simulink model "Cpchara"  (Simulink 7.4)
settings: Solver=ode45  StartTime=0.0  StopTime=100  RelTol=1e-3
libraries: simulink x3
settings Model: Creator=Balaji  LastModifiedBy=ss
settings DebuggingCC: StrictBusMsg=ErrorLevel1

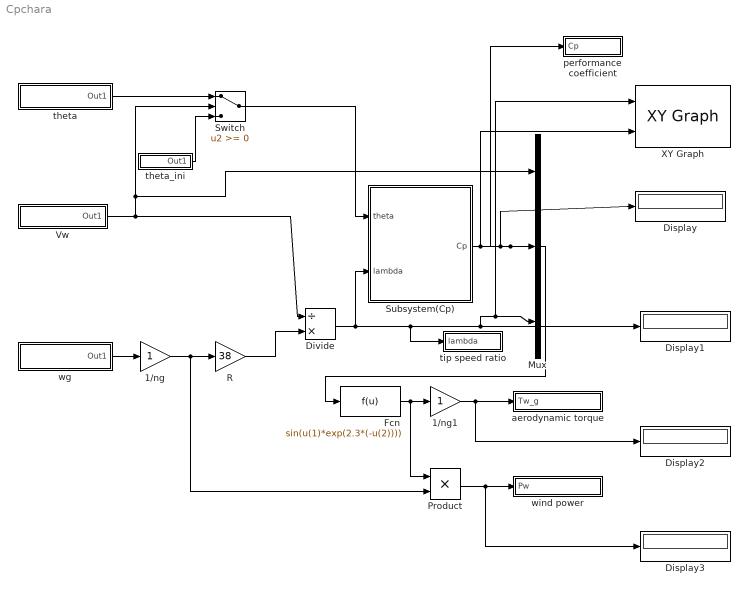
== system Cpchara ==
  1/ng : Gain  ParameterDataType=fixdt(1, 16)  ParameterScaling=2^0  OutDataType=fixdt(1, 16)  OutScaling=2^0
  1/ng1 : Gain  ParameterDataType=fixdt(1, 16)  ParameterScaling=2^0  OutDataType=fixdt(1, 16)  OutScaling=2^0
  Display{,1..3} (4 alike) : Display
  Divide : Product  Inputs=/*  OutDataType=fixdt(1, 16)  OutScaling=2^-10
  Fcn : Fcn  Expr=sin(u(1)*exp(2.3*(-u(2))))
  Mux : Mux  Inputs=3
  Product : Product  OutDataType=fixdt(1, 16)  OutScaling=2^0  RndMeth=Zero
  R : Gain  Gain=38  ParameterDataType=fixdt(1, 16)  ParameterScaling=2^0  OutDataType=fixdt(1, 16)  OutScaling=2^0
  Subsystem(Cp) : Subsystem
  Switch : Switch  OutDataType=fixdt(1, 16)  OutScaling=2^0  SampleTime=5
  Vw : Subsystem
  XY Graph : simulink/Sinks/XY Graph  SystemSampleTime=-1  xmin=2  xmax=16  ymin=0  ymax=0.5  st=0.05
  aerodynamic torque : Subsystem
  performance coefficient : Subsystem
  theta : Subsystem
  theta_ini : Subsystem
  tip speed ratio : Subsystem
  wg : Subsystem
  wind power : Subsystem
  wires:
  wg/1(Out1) -> 1/ng/1
  1/ng/1 -> R/1, Product/2
  Vw/1(Out1) -> Divide/1, Switch/2, Mux/1
  R/1 -> Divide/2
  theta/1(Out1) -> Switch/1
  theta_ini/1(Out1) -> Switch/3
  Switch/1 -> Subsystem(Cp)/1(theta)
  Divide/1 -> tip speed ratio/1(lambda), Display1/1, Mux/3, XY Graph/1, Subsystem(Cp)/2(lambda)
  Mux/1 -> Fcn/1
  Fcn/1 -> 1/ng1/1, Product/1
  1/ng1/1 -> aerodynamic torque/1(Tw_g), Display2/1
  Product/1 -> Display3/1, wind power/1(Pw)
  Subsystem(Cp)/1(Cp) -> Display/1, performance coefficient/1(Cp), Mux/2, XY Graph/2

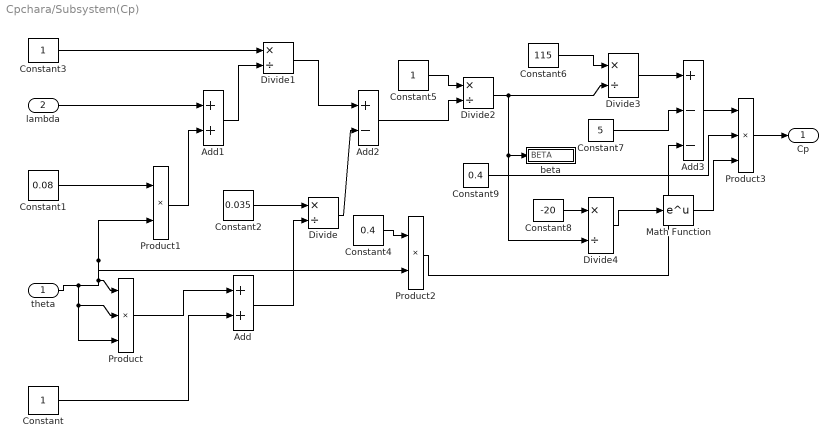
== system Cpchara/Subsystem(Cp) ==
  theta : Inport  OutDataType=fixdt(1, 16)  OutScaling=2^0
  lambda : Inport  Port=2  OutDataType=fixdt(1, 16)  OutScaling=2^0
  Add : Sum  OutDataType=fixdt(1, 16)  OutScaling=2^-10
  Add1 : Sum  OutDataType=fixdt(1, 16)  OutScaling=2^-10
  Add2 : Sum  Inputs=+-  OutDataType=fixdt(1, 16)  OutScaling=2^-10
  Add3 : Sum  Inputs=+--  OutDataType=fixdt(1, 16)  OutScaling=2^-10
  Constant : Constant  OutDataType=fixdt(1, 16)  OutScaling=2^0
  Constant1 : Constant  Value=0.08  OutDataType=fixdt(1, 16)  OutScaling=2^0
  Constant2 : Constant  Value=0.035  OutDataType=fixdt(1, 16)  OutScaling=2^0
  Constant3 : Constant  OutDataType=fixdt(1, 16)  OutScaling=2^0
  Constant4 : Constant  Value=0.4  OutDataType=fixdt(1, 16)  OutScaling=2^0
  Constant5 : Constant  OutDataType=fixdt(1, 16)  OutScaling=2^0
  Constant6 : Constant  Value=115  OutDataType=fixdt(1, 16)  OutScaling=2^0
  Constant7 : Constant  Value=5  OutDataType=fixdt(1, 16)  OutScaling=2^0
  Constant8 : Constant  Value=-20  OutDataType=fixdt(1, 16)  OutScaling=2^0
  Constant9 : Constant  Value=0.4  OutDataType=fixdt(1, 16)  OutScaling=2^0
  Divide{,1..4} (5 alike) : Product  Inputs=*/  OutDataType=fixdt(1, 16)  OutScaling=2^-10
  Math Function : Math  OutDataType=fixdt(1, 16)  OutScaling=2^0  SaturateOnIntegerOverflow=on
  Product : Product  Inputs=3  OutDataType=fixdt(1, 16)  OutScaling=2^0  RndMeth=Zero
  Product1 : Product  OutDataType=fixdt(1, 16)  OutScaling=2^0  RndMeth=Zero
  Product2 : Product  OutDataType=fixdt(1, 16)  OutScaling=2^0  RndMeth=Zero
  Product3 : Product  Inputs=3  OutDataType=fixdt(1, 16)  OutScaling=2^0  RndMeth=Zero
  beta : Subsystem
  Cp : Outport  OutDataType=fixdt(1, 16)  OutScaling=2^0
  wires:
  theta/1 -> Product/2, Product/3, Product/1, Product1/2, Product2/2
  Product/1 -> Add/1
  Constant/1 -> Add/2
  Constant1/1 -> Product1/1
  lambda/1 -> Add1/1
  Product1/1 -> Add1/2
  Constant2/1 -> Divide/1
  Add/1 -> Divide/2
  Constant3/1 -> Divide1/1
  Add1/1 -> Divide1/2
  Divide1/1 -> Add2/1
  Divide/1 -> Add2/2
  Constant4/1 -> Product2/1
  Constant5/1 -> Divide2/1
  Add2/1 -> Divide2/2
  Constant6/1 -> Divide3/1
  Divide2/1 -> Divide3/2, Divide4/2, beta/1(BETA)
  Divide3/1 -> Add3/1
  Constant7/1 -> Add3/2
  Product2/1 -> Add3/3
  Constant8/1 -> Divide4/1
  Divide4/1 -> Math Function/1
  Add3/1 -> Product3/1
  Constant9/1 -> Product3/2
  Math Function/1 -> Product3/3
  Product3/1 -> Cp/1

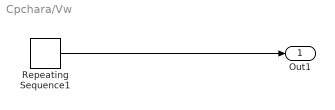
== system Cpchara/Vw ==
  Repeating Sequence1 : simulink/Sources/Repeating Sequence  SystemSampleTime=-1  rep_seq_t=[2 16]  rep_seq_y=[5.1775 41.42]
  Out1 : Outport  OutDataType=fixdt(1, 16)  OutScaling=2^0
  wires:
  Repeating Sequence1/1 -> Out1/1

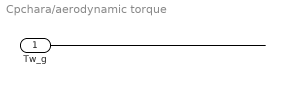
== system Cpchara/aerodynamic torque ==
  Tw_g : Inport  OutDataType=fixdt(1, 16)  OutScaling=2^0
  wires:
  Tw_g/1 -> ?

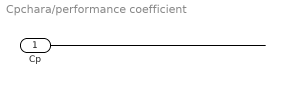
== system Cpchara/performance coefficient ==
  Cp : Inport  OutDataType=fixdt(1, 16)  OutScaling=2^0
  wires:
  Cp/1 -> ?

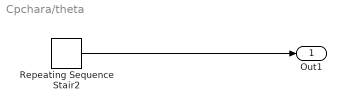
== system Cpchara/theta ==
  Repeating Sequence Stair2 : simulink/Sources/Repeating Sequence Stair  SystemSampleTime=-1  OutValues=[0 5 10 15 20 25 30 35 40 45]  tsamp=20  OutMin=[]  OutMax=[]  OutDataTypeStr=double  OutputDataTypeScalingMode=double  OutDataType=fixdt(0,8)  ConRadixGroup=Best Precision: Vector-wise  OutScaling=2^-12
  Out1 : Outport  OutDataType=fixdt(1, 16)  OutScaling=2^0
  wires:
  Repeating Sequence Stair2/1 -> Out1/1

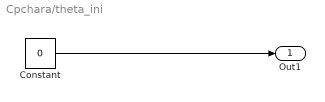
== system Cpchara/theta_ini ==
  Constant : Constant  Value=0  OutDataType=fixdt(1, 16)  OutScaling=2^0
  Out1 : Outport  OutDataType=fixdt(1, 16)  OutScaling=2^0
  wires:
  Constant/1 -> Out1/1

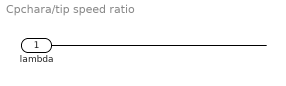
== system Cpchara/tip speed ratio ==
  lambda : Inport  OutDataType=fixdt(1, 16)  OutScaling=2^0
  wires:
  lambda/1 -> ?

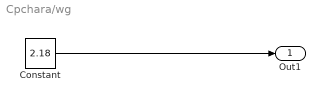
== system Cpchara/wg ==
  Constant : Constant  Value=2.18  OutDataType=fixdt(1, 16)  OutScaling=2^0
  Out1 : Outport  OutDataType=fixdt(1, 16)  OutScaling=2^0
  wires:
  Constant/1 -> Out1/1

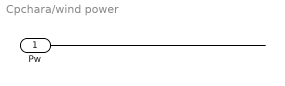
== system Cpchara/wind power ==
  Pw : Inport  OutDataType=fixdt(1, 16)  OutScaling=2^0
  wires:
  Pw/1 -> ?

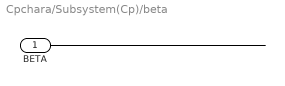
== system Cpchara/Subsystem(Cp)/beta ==
  BETA : Inport  OutDataType=fixdt(1, 16)  OutScaling=2^0
  wires:
  BETA/1 -> ?
